simulink model "MEGA2560hex_IOtask"  (Simulink 7.0)
undefined symbols (not defined in the file): Double, F64
libraries: logiclib x34, mathlib x28, REXduino_library x4, arclib x3, genlib x1
settings Model: Creator=Jarda  LastModifiedBy=Jarda  ExtModeTrigMode=oneshot  ExtModeArmWhenConnect=off

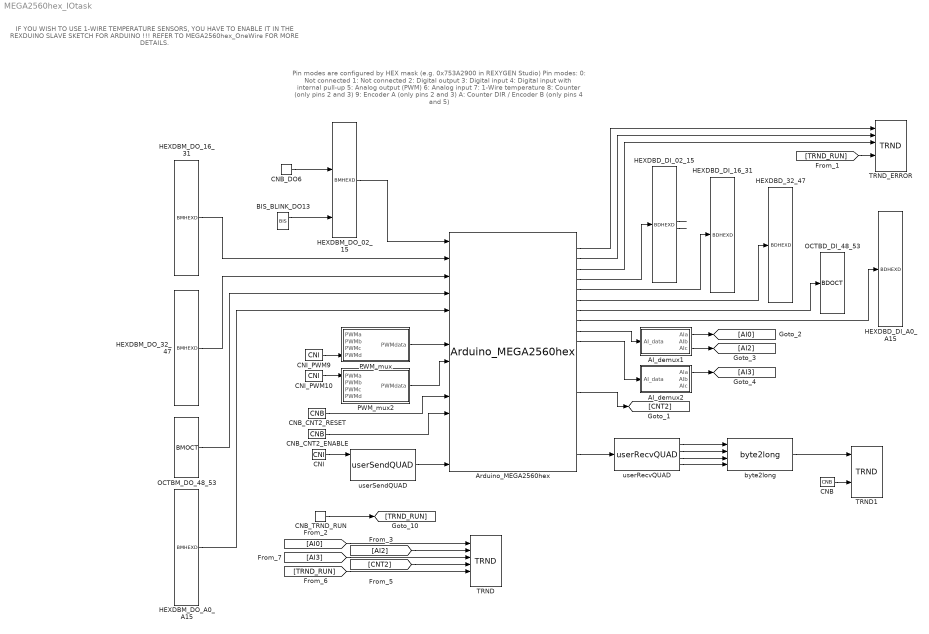
== system MEGA2560hex_IOtask ==
  note: Pin modes are configured by HEX mask
      |    (e.g. 0x753A2900 in REXYGEN Studio)
      |
      | Pin modes:
      | 0: Not connected
      | 1: Not connected
      | 2: Digital output
      | 3: Digital input
      | 4: Digital input with internal pull-up
      | 5: Analog output (PWM)
      | 6: Analog input
      | 7: 1-Wire temperature
      | 8: Counter (only pins 2 and 3)
      | 9: Encoder A (only pins 2 and 3)
      | A: Counter DIR / Encoder B (only pins 4 and 5)
  note: IF YOU WISH TO USE 1-WIRE TEMPERATURE
      | SENSORS, YOU HAVE TO ENABLE IT IN THE
      | REXDUINO SLAVE SKETCH FOR ARDUINO !!!
      |
      | REFER TO MEGA2560hex_OneWire FOR
      | MORE DETAILS.
  AI_demux1 : Subsystem
      mask Type: REX sequence
  AI_demux2 : Subsystem
      mask Type: REX sequence
  Arduino_MEGA2560hex : REXduino_library/Arduino_MEGA2560hex  comPort=/dev/ttyACM0  pinmodes_00_07=0x320A0800  pinmodes_08_15=0x00200554  pinmodes_16_23=0  pinmodes_24_31=0  pinmodes_32_39=0  pinmodes_40_47=0  pinmodes_48_53=0  pinmodes_A0_A7=0x00006606  pinmodes_A8_A15=0  usercmd=2: Four bytes
  BIS_BLINK_DO13 : genlib/BIS  Y0=off  t1=2  t2=4  t3=0  t4=4  t5=5  t6=6  t7=7  t8=8  RPT=on
  CNB : mathlib/CNB  YCN=on
  CNB_CNT2_ENABLE : mathlib/CNB  YCN=on
  CNB_CNT2_RESET : mathlib/CNB  YCN=off
  CNB_DO6 : mathlib/CNB  YCN=on
  CNB_TRND_RUN : mathlib/CNB  YCN=on
  CNI : mathlib/CNI  icn=1
  CNI_PWM10 : mathlib/CNI  icn=128
  CNI_PWM9 : mathlib/CNI  icn=128
  HEXDBD_32_47 : logiclib/BDHEXD  shift=0
  HEXDBD_DI_02_15 : logiclib/BDHEXD  shift=0
  HEXDBD_DI_16_31 : logiclib/BDHEXD  shift=0
  HEXDBD_DI_A0_A15 : logiclib/BDHEXD  shift=0
  HEXDBM_DO_02_15 : logiclib/BMHEXD  shift=0
  HEXDBM_DO_16_31 : logiclib/BMHEXD  shift=0
  HEXDBM_DO_32_47 : logiclib/BMHEXD  shift=0
  HEXDBM_DO_A0_A15 : logiclib/BMHEXD  shift=0
  OCTBD_DI_48_53 : logiclib/BDOCT  shift=0
  OCTBM_DO_48_53 : logiclib/BMOCT  shift=0
  PWM_mux : Subsystem
      mask Type: REX sequence
  PWM_mux2 : Subsystem
      mask Type: REX sequence
  TRND : arclib/TRND  n=4  l=14400  btype=8: Double  ptype1=1: Store  ptype2=1: Store  ptype3=1: Store  ptype4=1: Store  pfac=1  afac=0  arc=0  id=1  Title=Data trend  timesrc=1
  TRND1 : arclib/TRND  n=4  l=1000  btype=8: Double (F64)  ptype1=1: Store  ptype2=1: Store  ptype3=1: Store  ptype4=1: Store  pfac=1  afac=0  arc=0  id=0  Title=Trend Title  timesrc=1: CORETIMER
  TRND_ERROR : arclib/TRND  n=4  l=1000  btype=8: Double  ptype1=1: Store  ptype2=1: Store  ptype3=1: Store  ptype4=1: Store  pfac=1  afac=0  arc=0  id=1  Title=ERROR trend  timesrc=1
  byte2long : REXduino_library/byte2long
      mask Type: REX sequence
  userRecvQUAD : REXduino_library/userRecvQUAD
      mask Type: REX sequence
  userSendQUAD : REXduino_library/userSendQUAD
      mask Type: REX sequence
  wires:
  AI_demux1/1(AIa) -> [AI0]
  AI_demux1/3(AIc) -> [AI2]
  AI_demux2/1(AIa) -> [AI3]
  Arduino_MEGA2560hex/1 -> TRND_ERROR/1
  Arduino_MEGA2560hex/2 -> TRND_ERROR/2
  Arduino_MEGA2560hex/3 -> TRND_ERROR/3
  Arduino_MEGA2560hex/4 -> HEXDBD_DI_02_15/1
  Arduino_MEGA2560hex/5 -> HEXDBD_DI_16_31/1
  Arduino_MEGA2560hex/6 -> HEXDBD_32_47/1
  Arduino_MEGA2560hex/7 -> OCTBD_DI_48_53/1
  Arduino_MEGA2560hex/8 -> HEXDBD_DI_A0_A15/1
  Arduino_MEGA2560hex/9 -> AI_demux1/1(AI_data)
  Arduino_MEGA2560hex/10 -> AI_demux2/1(AI_data)
  Arduino_MEGA2560hex/15 -> [CNT2]
  Arduino_MEGA2560hex/21 -> userRecvQUAD/1
  BIS_BLINK_DO13/1 -> HEXDBM_DO_02_15/14
  CNB/1 -> TRND1/5
  CNB_CNT2_ENABLE/1 -> Arduino_MEGA2560hex/11
  CNB_CNT2_RESET/1 -> Arduino_MEGA2560hex/10
  CNB_DO6/1 -> HEXDBM_DO_02_15/7
  CNB_TRND_RUN/1 -> [TRND_RUN]
  CNI/1 -> userSendQUAD/1
  CNI_PWM10/1 -> PWM_mux2/1(PWMa)
  CNI_PWM9/1 -> PWM_mux/4(PWMd)
  [TRND_RUN] -> TRND_ERROR/5
  [AI0] -> TRND/1
  [AI2] -> TRND/2
  [CNT2] -> TRND/4
  [TRND_RUN] -> TRND/5
  [AI3] -> TRND/3
  HEXDBD_DI_02_15/8 -> ?
  HEXDBD_DI_02_15/9 -> ?
  HEXDBM_DO_02_15/1 -> Arduino_MEGA2560hex/1
  HEXDBM_DO_16_31/1 -> Arduino_MEGA2560hex/2
  HEXDBM_DO_32_47/1 -> Arduino_MEGA2560hex/3
  HEXDBM_DO_A0_A15/1 -> Arduino_MEGA2560hex/5
  OCTBM_DO_48_53/1 -> Arduino_MEGA2560hex/4
  PWM_mux/1(PWMdata) -> Arduino_MEGA2560hex/7
  PWM_mux2/1(PWMdata) -> Arduino_MEGA2560hex/8
  byte2long/1 -> TRND1/1
  userRecvQUAD/1 -> byte2long/1
  userRecvQUAD/2 -> byte2long/2
  userRecvQUAD/3 -> byte2long/3
  userRecvQUAD/4 -> byte2long/4
  userSendQUAD/1 -> Arduino_MEGA2560hex/14

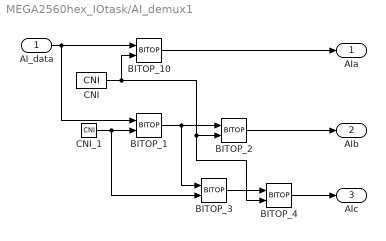
== system MEGA2560hex_IOtask/AI_demux1 ==
  AI_data : Inport  Port=1
  BITOP_1 : logiclib/BITOP  iop=6: Shift Right
  BITOP_10 : logiclib/BITOP  iop=3: Bit AND
  BITOP_2 : logiclib/BITOP  iop=3: Bit AND
  BITOP_3 : logiclib/BITOP  iop=6: Shift Right
  BITOP_4 : logiclib/BITOP  iop=3: Bit AND
  CNI : mathlib/CNI  icn=1023
  CNI_1 : mathlib/CNI  icn=10
  AIa : Outport  Port=1
  AIb : Outport  Port=2
  AIc : Outport  Port=3
  wires:
  AI_data/1 -> BITOP_1/1, BITOP_10/1
  BITOP_1/1 -> BITOP_2/1, BITOP_3/1
  BITOP_10/1 -> AIa/1
  BITOP_2/1 -> AIb/1
  BITOP_3/1 -> BITOP_4/1
  BITOP_4/1 -> AIc/1
  CNI/1 -> BITOP_10/2, BITOP_2/2, BITOP_4/2
  CNI_1/1 -> BITOP_1/2, BITOP_3/2

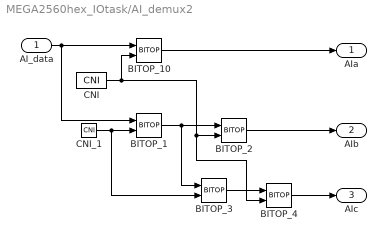
== system MEGA2560hex_IOtask/AI_demux2 ==
  AI_data : Inport  Port=1
  BITOP_1 : logiclib/BITOP  iop=6: Shift Right
  BITOP_10 : logiclib/BITOP  iop=3: Bit AND
  BITOP_2 : logiclib/BITOP  iop=3: Bit AND
  BITOP_3 : logiclib/BITOP  iop=6: Shift Right
  BITOP_4 : logiclib/BITOP  iop=3: Bit AND
  CNI : mathlib/CNI  icn=1023
  CNI_1 : mathlib/CNI  icn=10
  AIa : Outport  Port=1
  AIb : Outport  Port=2
  AIc : Outport  Port=3
  wires:
  AI_data/1 -> BITOP_1/1, BITOP_10/1
  BITOP_1/1 -> BITOP_2/1, BITOP_3/1
  BITOP_10/1 -> AIa/1
  BITOP_2/1 -> AIb/1
  BITOP_3/1 -> BITOP_4/1
  BITOP_4/1 -> AIc/1
  CNI/1 -> BITOP_10/2, BITOP_2/2, BITOP_4/2
  CNI_1/1 -> BITOP_1/2, BITOP_3/2

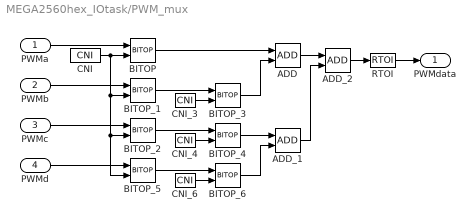
== system MEGA2560hex_IOtask/PWM_mux ==
  PWMa : Inport  Port=1
  PWMb : Inport  Port=2
  PWMc : Inport  Port=3
  PWMd : Inport  Port=4
  ADD : mathlib/ADD
  ADD_1 : mathlib/ADD
  ADD_2 : mathlib/ADD
  BITOP : logiclib/BITOP  iop=3: Bit AND
  BITOP_1 : logiclib/BITOP  iop=3: Bit AND
  BITOP_2 : logiclib/BITOP  iop=3: Bit AND
  BITOP_3 : logiclib/BITOP  iop=5: Shift Left
  BITOP_4 : logiclib/BITOP  iop=5: Shift Left
  BITOP_5 : logiclib/BITOP  iop=3: Bit AND
  BITOP_6 : logiclib/BITOP  iop=5: Shift Left
  CNI : mathlib/CNI  icn=255
  CNI_3 : mathlib/CNI  icn=8
  CNI_4 : mathlib/CNI  icn=16
  CNI_6 : mathlib/CNI  icn=24
  RTOI : mathlib/RTOI
  PWMdata : Outport  Port=1
  wires:
  ADD/1 -> ADD_2/1
  ADD_1/1 -> ADD_2/2
  ADD_2/1 -> RTOI/1
  BITOP/1 -> ADD/1
  BITOP_1/1 -> BITOP_3/1
  BITOP_2/1 -> BITOP_4/1
  BITOP_3/1 -> ADD/2
  BITOP_4/1 -> ADD_1/1
  BITOP_5/1 -> BITOP_6/1
  BITOP_6/1 -> ADD_1/2
  CNI/1 -> BITOP/2, BITOP_1/2, BITOP_2/2, BITOP_5/2
  CNI_3/1 -> BITOP_3/2
  CNI_4/1 -> BITOP_4/2
  CNI_6/1 -> BITOP_6/2
  PWMa/1 -> BITOP/1
  PWMb/1 -> BITOP_1/1
  PWMc/1 -> BITOP_2/1
  PWMd/1 -> BITOP_5/1
  RTOI/1 -> PWMdata/1

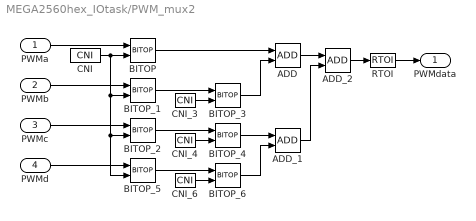
== system MEGA2560hex_IOtask/PWM_mux2 ==
  PWMa : Inport  Port=1
  PWMb : Inport  Port=2
  PWMc : Inport  Port=3
  PWMd : Inport  Port=4
  ADD : mathlib/ADD
  ADD_1 : mathlib/ADD
  ADD_2 : mathlib/ADD
  BITOP : logiclib/BITOP  iop=3: Bit AND
  BITOP_1 : logiclib/BITOP  iop=3: Bit AND
  BITOP_2 : logiclib/BITOP  iop=3: Bit AND
  BITOP_3 : logiclib/BITOP  iop=5: Shift Left
  BITOP_4 : logiclib/BITOP  iop=5: Shift Left
  BITOP_5 : logiclib/BITOP  iop=3: Bit AND
  BITOP_6 : logiclib/BITOP  iop=5: Shift Left
  CNI : mathlib/CNI  icn=255
  CNI_3 : mathlib/CNI  icn=8
  CNI_4 : mathlib/CNI  icn=16
  CNI_6 : mathlib/CNI  icn=24
  RTOI : mathlib/RTOI
  PWMdata : Outport  Port=1
  wires:
  ADD/1 -> ADD_2/1
  ADD_1/1 -> ADD_2/2
  ADD_2/1 -> RTOI/1
  BITOP/1 -> ADD/1
  BITOP_1/1 -> BITOP_3/1
  BITOP_2/1 -> BITOP_4/1
  BITOP_3/1 -> ADD/2
  BITOP_4/1 -> ADD_1/1
  BITOP_5/1 -> BITOP_6/1
  BITOP_6/1 -> ADD_1/2
  CNI/1 -> BITOP/2, BITOP_1/2, BITOP_2/2, BITOP_5/2
  CNI_3/1 -> BITOP_3/2
  CNI_4/1 -> BITOP_4/2
  CNI_6/1 -> BITOP_6/2
  PWMa/1 -> BITOP/1
  PWMb/1 -> BITOP_1/1
  PWMc/1 -> BITOP_2/1
  PWMd/1 -> BITOP_5/1
  RTOI/1 -> PWMdata/1
